simulink library "LIBRARY_SAD"  (R2025b)
settings: Solver=VariableStepAuto  StartTime=0.0  StopTime=10.0  RelTol=1e-3
values from neighbouring files (symbols this model uses):
  c = astroConstants(5)*1e3    [SCRIPT_SAD_DEMO.m]    (also in lab_7.m)
  eps_E = deg2rad(astroConstants(63))    [SCRIPT_SAD_DEMO.m]    (also in lab_7.m)
  F0 = 237    [SCRIPT_SAD_DEMO.m]
  F_e = 1358    [SCRIPT_SAD_DEMO.m]    (also in lab_7.m)
  g0_1 = -29404.8e-9    (= -2.94048e-05)    [lab_7.m]
  g1_1 = -1450.9e-9    (= -1.4509e-06)    [lab_7.m]
  h1_1 = 4652.5e-9    (= 4.6525e-06)    [lab_7.m]
  j_B = [0.01; 0.05; 0.01]    [SCRIPT_SAD_DEMO.m]    (also in lab_7.m)
  mu = astroConstants(13)    [SCRIPT_SAD_DEMO.m]    (also in lab_7.m)
  n = sqrt( (mu/ (a)^3))    [SCRIPT_SAD_DEMO.m]    (also in lab_7.m = sqrt((mu/ ((a/1000)^3))))
  n_sun = 2*pi/T_sun    (= 1.99238499086e-07)    [SCRIPT_SAD_DEMO.m]    (also in lab_7.m)
  r_sun = 1*ua    [SCRIPT_SAD_DEMO.m]    (also in lab_7.m)
  Re = astroConstants(23)    [SCRIPT_SAD_DEMO.m]    (also in lab_7.m)
  theta = 0    [SCRIPT_SAD_DEMO.m]    (also in lab_7.m)
  w0 = [0; 0; n]    [SCRIPT_SAD_DEMO.m]    (also in lab_7.m)
  w_E = deg2rad(15.04)/3600    [SCRIPT_SAD_DEMO.m]    (also in lab_7.m)
undefined symbols (not defined in the file or in its folder): Ix, Iy, Iz, phi0, psi0, SRP, theta0
libraries: matrix_library x13, lIBRARY_SAD_SAD x12, $bdroot x3, LIBRARY_SAD_SAD x3, simulink x1
(part 2 of 2)

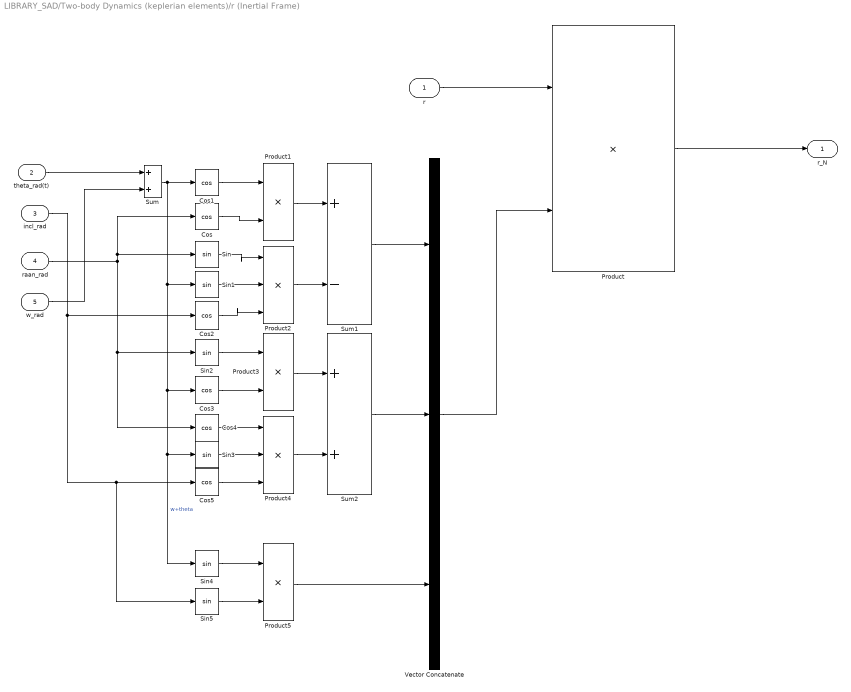
== system LIBRARY_SAD/Two-body Dynamics (keplerian elements)/r (Inertial Frame) ==
  r : Inport
  theta_rad(t) : Inport  Port=2
  incl_rad : Inport  Port=3
  raan_rad : Inport  Port=4
  w_rad : Inport  Port=5
  Cos{,1..5} (6 alike) : Trigonometry  Operator=cos
  Product{,1,3,5} (4 alike) : Product
  Product2 : Product  Inputs=3
  Product4 : Product  Inputs=3
  Sin{,1..5} (6 alike) : Trigonometry
  Sum : Sum
  Sum1 : Sum  Inputs=+-
  Sum2 : Sum
  Vector Concatenate : Concatenate  NumInputs=3
  r_N : Outport
  wires:
  r/1 -> Product/1
  raan_rad/1 -> Cos/1, Sin/1, Cos4/1, Sin2/1
  w_rad/1 -> Sum/2
  Cos/1 -> Product1/2
  theta_rad(t)/1 -> Sum/1
  Sum/1 -> Sin4/1, Sin3/1, Cos3/1, Sin1/1, Cos1/1  "w+theta"
  Cos1/1 -> Product1/1
  Product1/1 -> Sum1/1
  Product2/1 -> Sum1/2
  Sin/1 -> Product2/1
  Sin1/1 -> Product2/2
  Cos2/1 -> Product2/3
  incl_rad/1 -> Sin5/1, Cos5/1, Cos2/1
  Sum1/1 -> Vector Concatenate/1
  Sum2/1 -> Vector Concatenate/2
  Sin2/1 -> Product3/1
  Cos3/1 -> Product3/2
  Product3/1 -> Sum2/1
  Product4/1 -> Sum2/2
  Cos4/1 -> Product4/1
  Sin3/1 -> Product4/2
  Cos5/1 -> Product4/3
  Sin4/1 -> Product5/1
  Sin5/1 -> Product5/2
  Product5/1 -> Vector Concatenate/3
  Vector Concatenate/1 -> Product/2
  Product/1 -> r_N/1

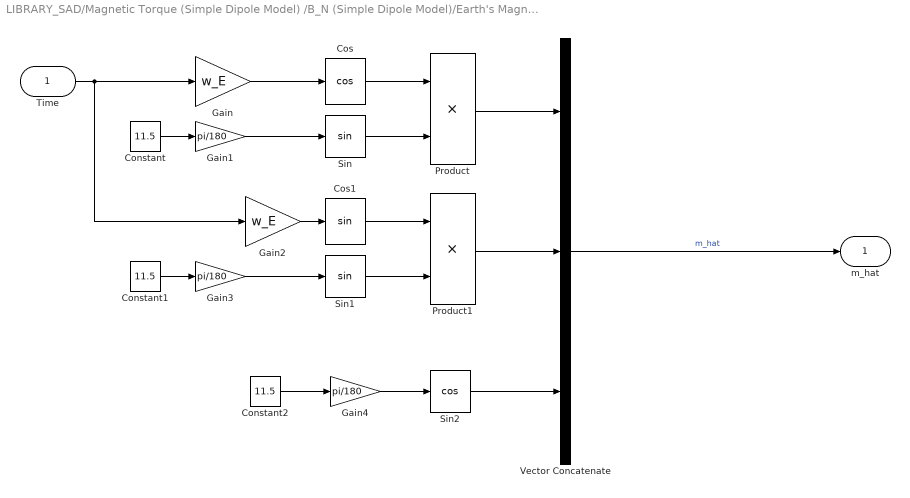
== system LIBRARY_SAD/Magnetic Torque (Simple Dipole Model) /B_N (Simple Dipole Model)/Earth's Magnetic Dipole (unit vector) ==
  Time : Inport
  Constant : Constant  Value=11.5
  Constant1 : Constant  Value=11.5
  Constant2 : Constant  Value=11.5
  Cos : Trigonometry  Operator=cos
  Cos1 : Trigonometry
  Gain : Gain  Gain=w_E
  Gain1 : Gain  Gain=pi/180
  Gain2 : Gain  Gain=w_E
  Gain3 : Gain  Gain=pi/180
  Gain4 : Gain  Gain=pi/180
  Product : Product
  Product1 : Product
  Sin : Trigonometry
  Sin1 : Trigonometry
  Sin2 : Trigonometry  Operator=cos
  Vector Concatenate : Concatenate  NumInputs=3
  m_hat : Outport
  wires:
  Gain/1 -> Cos/1
  Cos/1 -> Product/1
  Sin/1 -> Product/2
  Constant/1 -> Gain1/1
  Gain1/1 -> Sin/1
  Product/1 -> Vector Concatenate/1
  Product1/1 -> Vector Concatenate/2
  Cos1/1 -> Product1/1
  Gain2/1 -> Cos1/1
  Time/1 -> Gain2/1, Gain/1
  Constant2/1 -> Gain4/1
  Gain4/1 -> Sin2/1
  Sin2/1 -> Vector Concatenate/3
  Vector Concatenate/1 -> m_hat/1  "m_hat"
  Gain3/1 -> Sin1/1
  Constant1/1 -> Gain3/1
  Sin1/1 -> Product1/2

== system LIBRARY_SAD/Magnetic Torque (Simple Dipole Model) /B_N (Simple Dipole Model)/H_0 ==
  Constant1 : Constant  Value=2
  Constant2 : Constant  Value=2
  Constant3 : Constant  Value=g0_1
  Constant4 : Constant  Value=g1_1
  Constant5 : Constant  Value=2
  Constant6 : Constant  Value=h1_1
  Power : Math  Operator=pow
  Power1 : Math  Operator=pow
  Power2 : Math  Operator=pow
  Sqrt : Sqrt
  Sum : Sum  Inputs=+++
  H_0 : Outport
  wires:
  Constant3/1 -> Power/1
  Power2/1 -> Sum/3
  Power1/1 -> Sum/2
  Sqrt/1 -> H_0/1
  Power/1 -> Sum/1
  Sum/1 -> Sqrt/1
  Constant1/1 -> Power/2
  Constant2/1 -> Power1/2
  Constant4/1 -> Power1/1
  Constant6/1 -> Power2/1
  Constant5/1 -> Power2/2
